simulink model "DC_Motor"  (R2023a)
settings: Solver=VariableStepAuto  StartTime=0.0  StopTime=10.0  RelTol=1e-3
values from neighbouring files (symbols this model uses):
  a = 1.525    [AllePlots_aus_UEF.m]    (also in DC_Motor_param.m = 2.45e-06; PT2.m = 4; Polynomfit_for_students.m = fitvariables(1,1); systemcharakter.m = 1)
  J = 44.2*10^-7    (= 4.42e-06)    [DC_Motor_param.m]
  Km = 38*10^-3    (= 0.038)    [DC_Motor_param.m]
  Kn = 250/60*(2*pi)    (= 26.1799387799)    [DC_Motor_param.m]
  L = 1.04*10^-3    (= 0.00104)    [DC_Motor_param.m]
  R = 7.03    [DC_Motor_param.m]
settings Model: Creator=Samuel Huser  LastModifiedBy=Samuel Huser

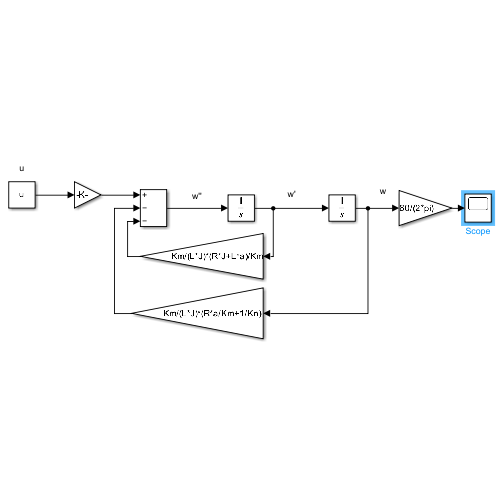
[thumbnail: Simulink's stored preview of the top-level diagram]
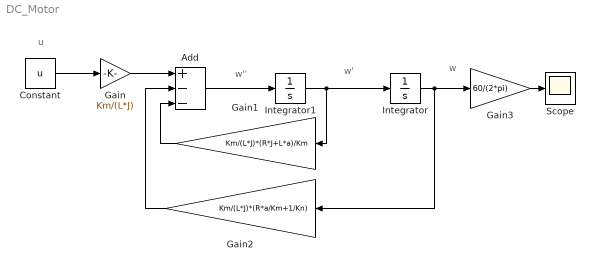
== system DC_Motor ==
  note: w
  note: w'
  note: u
  note: w''
  Add : Sum  Inputs=+--
  Constant : Constant  Value=u
  Gain : Gain  Gain=Km/(L*J)
  Gain1 : Gain  Gain=Km/(L*J)*(R*J+L*a)/Km
  Gain2 : Gain  Gain=Km/(L*J)*(R*a/Km+1/Kn)
  Gain3 : Gain  Gain=60/(2*pi)
  Integrator : Integrator
  Integrator1 : Integrator
  Scope : Scope
  wires:
  Integrator1/1 -> Integrator/1, Gain1/1
  Integrator/1 -> Gain2/1, Gain3/1
  Add/1 -> Integrator1/1
  Constant/1 -> Gain/1
  Gain/1 -> Add/1
  Gain2/1 -> Add/2
  Gain1/1 -> Add/3
  Gain3/1 -> Scope/1
